simulink model "sep_ekf_rover"  (R2024b)
settings: Solver=FixedStepDiscrete  StartTime=0  StopTime=100  FixedStep=0.02  RelTol=1e-3
settings Model: Creator=Usuario  LastModifiedBy=Usuario

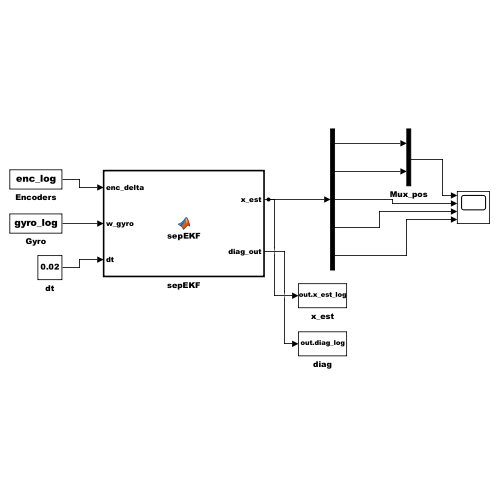
[thumbnail: Simulink's stored preview of the top-level diagram]
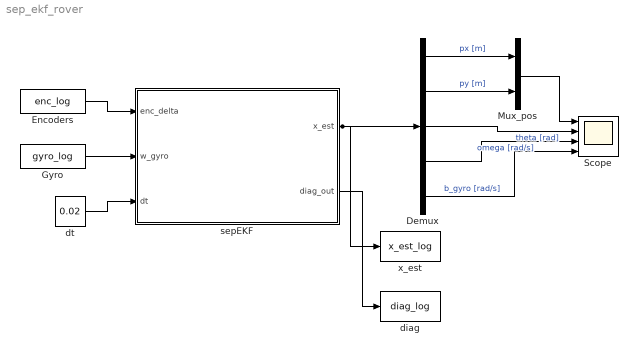
== system sep_ekf_rover ==
  Demux : Demux  Outputs=5
  Encoders : FromWorkspace  VariableName=enc_log  SampleTime=0.02  Interpolate=off  OutputAfterFinalValue=Setting to zero
  Gyro : FromWorkspace  VariableName=gyro_log  SampleTime=0.02  Interpolate=off  OutputAfterFinalValue=Holding final value
  Mux_pos : Mux  Inputs=2
  Scope : Scope  NumInputPorts=4
  diag : ToWorkspace  VariableName=diag_log  SaveFormat=Timeseries  SampleTime=0.02
  dt : Constant  Value=0.02  SampleTime=0.02
  sepEKF : MATLAB Function  TreatAsAtomicUnit=on
  x_est : ToWorkspace  VariableName=x_est_log  SaveFormat=Timeseries  SampleTime=0.02
  wires:
  Encoders/1 -> sepEKF/1(enc_delta)
  Gyro/1 -> sepEKF/2(w_gyro)
  Demux/3 -> Scope/2  "theta [rad]"
  Demux/1 -> Mux_pos/1  "px [m]"
  dt/1 -> sepEKF/3(dt)
  Demux/2 -> Mux_pos/2  "py [m]"
  sepEKF/1(x_est) -> x_est/1, Demux/1
  sepEKF/2(diag_out) -> diag/1
  Mux_pos/1 -> Scope/1
  Demux/4 -> Scope/3  "omega [rad/s]"
  Demux/5 -> Scope/4  "b_gyro [rad/s]"

== matlab function sep_ekf_rover/sepEKF ==
  data: enc_delta input; x_est output; w_gyro input; dt input; diag_out output
function [x_est, diag_out] = sepEKF(enc_delta, w_gyro, dt)
%#codegen
persistent x P
geo = sep_geo_params();
prm = sep_ekf_params();
if isempty(x)
    x = zeros(5,1);
    P = diag(prm.P0);
end
x_est = zeros(5,1);
diag_out = zeros(3,1);
[ds, dth, moving, ~] = sep_odometry(enc_delta(:), geo);
[x, P, xe, dg] = sep_ekf_step(x, P, ds, dth, w_gyro, dt, moving, prm);
x_est(:) = xe;
diag_out(:) = dg;
end
